simulink model "P5PIDModel"  (R2015b)
settings: Solver=VariableStepAuto  StartTime=0.0  StopTime=10.0  RelTol=1e-3
libraries: fuzblock x2
settings Model: Creator=Pepe  LastModifiedBy=Pepe

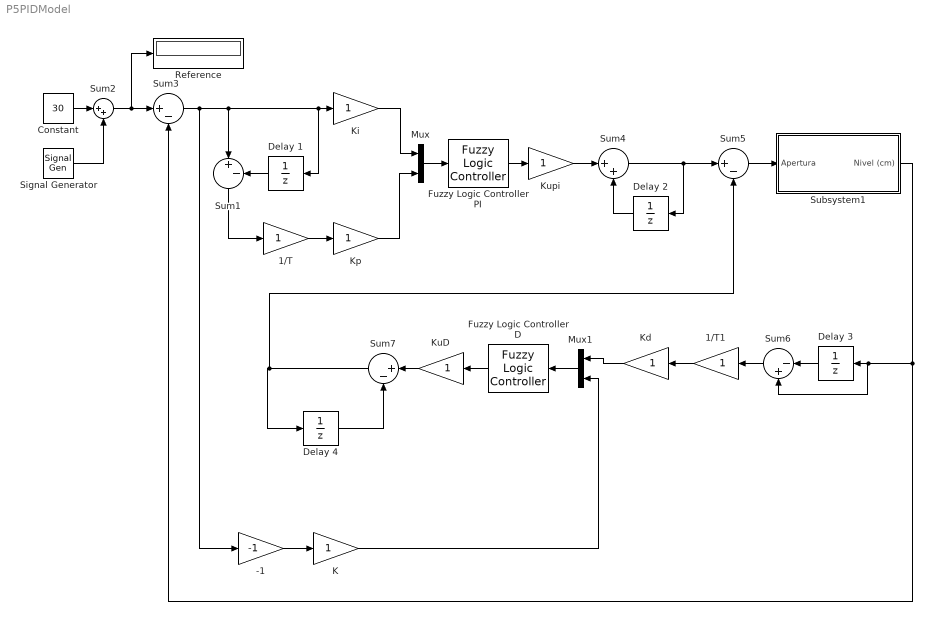
== system P5PIDModel ==
  -1 : Gain  Gain=-1  SaturateOnIntegerOverflow=on  OutDataTypeStr=Inherit: Same as input  ParamDataTypeStr=Inherit: Same as input
  1/T : Gain  SaturateOnIntegerOverflow=on  OutDataTypeStr=Inherit: Same as input  ParamDataTypeStr=Inherit: Same as input
  1/T1 : Gain  SaturateOnIntegerOverflow=on  OutDataTypeStr=Inherit: Same as input  ParamDataTypeStr=Inherit: Same as input
  Constant : Constant  Value=30
  Delay {1..4} (4 alike) : UnitDelay
  Fuzzy Logic Controller D : fuzblock/Fuzzy Logic  Controller  fis=[]
  Fuzzy Logic Controller PI : fuzblock/Fuzzy Logic  Controller  fis=[]
  K : Gain  SaturateOnIntegerOverflow=on  OutDataTypeStr=Inherit: Same as input  ParamDataTypeStr=Inherit: Same as input
  Kd : Gain  SaturateOnIntegerOverflow=on  OutDataTypeStr=Inherit: Same as input  ParamDataTypeStr=Inherit: Same as input
  Ki : Gain  SaturateOnIntegerOverflow=on  OutDataTypeStr=Inherit: Same as input  ParamDataTypeStr=Inherit: Same as input
  Kp : Gain  SaturateOnIntegerOverflow=on  OutDataTypeStr=Inherit: Same as input  ParamDataTypeStr=Inherit: Same as input
  KuD : Gain  SaturateOnIntegerOverflow=on  OutDataTypeStr=Inherit: Same as input  ParamDataTypeStr=Inherit: Same as input
  Kupi : Gain  SaturateOnIntegerOverflow=on  OutDataTypeStr=Inherit: Same as input  ParamDataTypeStr=Inherit: Same as input
  Mux : Mux  Inputs=2
  Mux1 : Mux  Inputs=2
  Reference : Display
  Signal Generator : SignalGenerator  WaveForm=square  Amplitude=10  Frequency=0.0001
  Subsystem1 : Subsystem
  Sum{1,3,5,7} (4 alike) : Sum  Inputs=|+-  SaturateOnIntegerOverflow=on  InputSameDT=on  OutDataTypeStr=Inherit: Same as first input
  Sum2 : Sum  Inputs=|++  SaturateOnIntegerOverflow=on  InputSameDT=on  OutDataTypeStr=Inherit: Same as first input
  Sum4 : Sum  Inputs=|++  SaturateOnIntegerOverflow=on  InputSameDT=on  OutDataTypeStr=Inherit: Same as first input
  Sum6 : Sum  Inputs=|-+  SaturateOnIntegerOverflow=on  InputSameDT=on  OutDataTypeStr=Inherit: Same as first input
  wires:
  Constant/1 -> Sum2/1
  Signal Generator/1 -> Sum2/2
  Sum2/1 -> Sum3/1, Reference/1
  Sum3/1 -> -1/1, Sum1/1, Delay 1/1, Ki/1
  Delay 1/1 -> Sum1/2
  Sum1/1 -> 1/T/1
  1/T/1 -> Kp/1
  Kp/1 -> Mux/2
  Ki/1 -> Mux/1
  Mux/1 -> Fuzzy Logic Controller PI/1
  Fuzzy Logic Controller PI/1 -> Kupi/1
  Kupi/1 -> Sum4/1
  Delay 2/1 -> Sum4/2
  Sum4/1 -> Sum5/1, Delay 2/1
  Sum5/1 -> Subsystem1/1(Apertura)
  Subsystem1/1(Nivel (cm)) -> Sum6/2, Delay 3/1, Sum3/2
  Delay 3/1 -> Sum6/1
  Sum6/1 -> 1/T1/1
  1/T1/1 -> Kd/1
  Mux1/1 -> Fuzzy Logic Controller D/1
  Kd/1 -> Mux1/1
  -1/1 -> K/1
  K/1 -> Mux1/2
  Fuzzy Logic Controller D/1 -> KuD/1
  KuD/1 -> Sum7/1
  Delay 4/1 -> Sum7/2
  Sum7/1 -> Sum5/2, Delay 4/1

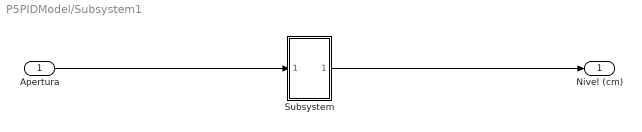
== system P5PIDModel/Subsystem1 ==
  Apertura : Inport
  Subsystem : Subsystem
  Nivel (cm) : Outport
  wires:
  Subsystem/1(Out1) -> Nivel (cm)/1
  Apertura/1 -> Subsystem/1(In1)

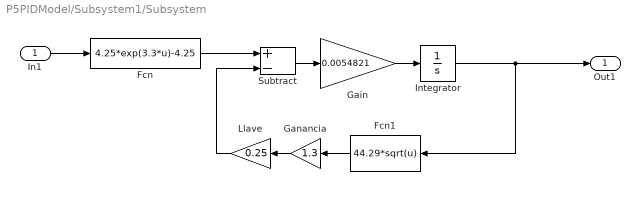
== system P5PIDModel/Subsystem1/Subsystem ==
  In1 : Inport
  Fcn : Fcn  Expr=4.25*exp(3.3*u)-4.25
  Fcn1 : Fcn  Expr=44.29*sqrt(u)
  Gain : Gain  Gain=0.0054821
  Ganancia : Gain  Gain=1.3
  Integrator : Integrator  InitialCondition=15  LimitOutput=on  UpperSaturationLimit=78  LowerSaturationLimit=0
  Llave : Gain  Gain=0.25
  Subtract : Sum  Inputs=+-
  Out1 : Outport
  wires:
  Llave/1 -> Subtract/2
  Fcn1/1 -> Ganancia/1
  Gain/1 -> Integrator/1
  Fcn/1 -> Subtract/1
  Ganancia/1 -> Llave/1
  Subtract/1 -> Gain/1
  In1/1 -> Fcn/1
  Integrator/1 -> Out1/1, Fcn1/1
